simulink model "MPSKimparfait"  (Simulink 10.1)
settings: Solver=VariableStepAuto  StartTime=0.0  StopTime=inf  RelTol=1e-3
undefined symbols (not defined in the file or in its folder): M
libraries: commdigbbndpm3 x2, commfilt2 x2, commchan3 x1, commsync2 x1, commsink2 x1, commutil2 x1, commrflib2 x1, commrandsrc3 x1, dspsigops x1
settings Model: Creator=iba  LastModifiedBy=iba
settings DataIOCC: SaveFormat=Dataset  ReturnWorkspaceOutputs=on
settings OptimizationCC: LifeSpan=auto
settings DebuggingCC: UnderspecifiedInitializationDetection=Simplified  MergeDetectMultiDrivingBlocksExec=error  SFUnexpectedBacktrackingDiag=error  SFNoUnconditionalDefaultTransitionDiag=error  SFExecutionAtInitializationDiag=warning  ArithmeticOperatorsInVariantConditions=error
settings HardwareCC: ProdBitPerPointer=64  ProdBitPerSizeT=64  ProdBitPerPtrDiffT=64  ProdLargestAtomicFloat=Float  ProdIntDivRoundTo=Zero  ProdEndianess=LittleEndian  ProdWordSize=64  ProdHWDeviceType=Intel->x86-64 (Windows64)
settings ModelReferenceCC: PropagateSignalLabelsOutOfModel=on
settings SFSimCC: SimUseLocalCustomCode=on  CustomCodeUndefinedFunction=FilterOut
settings RTWCC: RTWUseLocalCustomCode=on
settings CodeAppCC: StateflowObjectComments=off
settings GRTTargetCC: TargetLangStandard=C99 (ISO)  CombineOutputUpdateFcns=on  GRTInterface=off
settings ConfigComp: CovMetricSettings=dwe  CovHtmlReporting=off  CovSaveCumulativeToWorkspaceVar=off  CovSaveSingleToWorkspaceVar=off  CovExternalEMLEnable=on

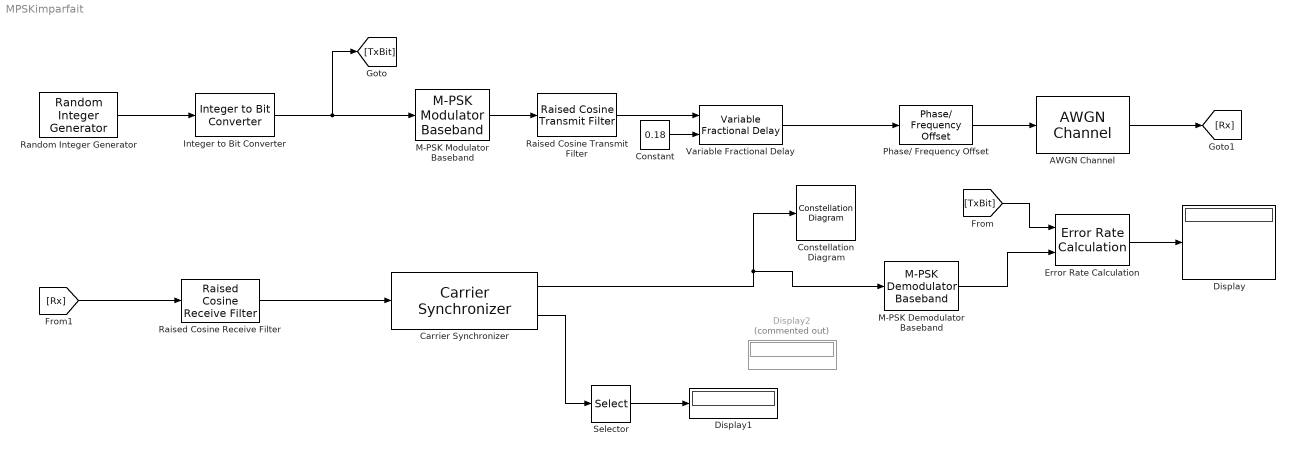
== system MPSKimparfait ==
  AWGN Channel : commchan3/AWGN Channel  InputProcessing=Columns as channels (frame based)  seed=67  noiseMode="Signal to noise ratio  (Eb/No)"  EbNodB=20  EsNodB=10  SNRdB=10  bitsPerSym=log2(M)  Ps=0.1  Tsym=1e-6  variance=1
  Carrier Synchronizer : commsync2/Carrier Synchronizer  Modulation=8PSK  ModulationPhaseOffset=Custom  CustomPhaseOffset=0  SamplesPerSymbol=1000  DampingFactor=0.701  NormalizedLoopBandwidth=0.0001  EstimatedPhaseErrorOutputPort=on  SimulateUsing=Code generation
  Constant : Constant  Value=0.18
  Constellation Diagram : ConstellationDiagram
  Display : Display
  Display1 : Display
  Display2 : Display  Commented=on
  Error Rate Calculation : commsink2/Error Rate Calculation  N=10*log2(M)  st_delay=0  cp_mode=Entire frame  subframe=[]  PMode=Port  WsName=MonTEB  RsMode2=off  stop=on  numErr=100  maxBits=1e6
  Integer to Bit Converter : commutil2/Integer to Bit Converter  nbits=log2(M)  signedInputValues=Unsigned  bitOrder=MSB first  outDtype=Inherit via internal rule
  M-PSK Demodulator Baseband : commdigbbndpm3/M-PSK Demodulator Baseband  M=M  OutType=Bit  DecType=Hard decision  VarSource=Dialog  Variance=1  Dec=Gray  Mapping=[0:7]  Ph=0  outDtype1=Inherit via internal rule  outDtype2=Inherit via internal rule  derotateFactorWordLen=16  derotateFactorDataTypeStr=Inherit: Same word length as input  derotateFactorLastDataTypeStr=Inherit: Same word length as input
  M-PSK Modulator Baseband : commdigbbndpm3/M-PSK Modulator Baseband  M=M  InType=Bit  Enc=Gray  Mapping=[0:7]  Ph=0  outDtype=double  outWordLen=16  outUDDataType=sfix(16)  outFracLenMode=Best precision  outFracLen=15  outDataTypeStr=double  outLastDataTypeStr=double
  Phase/ Frequency Offset : commrflib2/Phase// Frequency Offset  phaseOffset=18  freqPort=off  freqOffset=0
  Raised Cosine Receive Filter : commfilt2/Raised Cosine Receive Filter  filtType=Square root  R=0.7  filtSpan=10  N=10  downFactor=10  downOffset=0  filterGain=1  InputProcessing=Columns as channels (frame based)  RateOptions=Enforce single-rate processing  framing=Mute  checkCoeff=off  variableName=rcRxFilt  currentFiltSpan=10  D=(10)/2  inputOffset=0  sampMode=Mute  saveAsFlag=0  rateMode=Downsampling  checkGain=Normalized  launchFVT=on  roundingMode=Floor  overflowMode=off  coeffDataTypeStr=Inherit: Same word length as input  coeffMin=[]  coeffMax=[]  coeffLastDataTypeStr=Inherit: Same word length as input  accumDataTypeStr=Inherit: Same as product output  accumLastDataTypeStr=Inherit: Same as product output  outputDataTypeStr=Inherit: Same as accumulator  outputMin=[]  outputMax=[]  outputLastDataTypeStr=Inherit: Same as accumulator
  Raised Cosine Transmit Filter : commfilt2/Raised Cosine Transmit Filter  filtType=Square root  R=0.7  filtSpan=10  N=10  filterGain=1  InputProcessing=Columns as channels (frame based)  RateOptions=Enforce single-rate processing  framing=Mute  checkCoeff=off  variableName=rcTxFilt  checkGain=Normalized  sampMode=Mute  saveAsFlag=0  currentFiltSpan=10  D=5  launchFVT=on  roundingMode=Floor  overflowMode=off  coeffDataTypeStr=Inherit: Same word length as input  coeffMin=[]  coeffMax=[]  coeffLastDataTypeStr=Inherit: Same word length as input  outputDataTypeStr=Inherit: Same as accumulator  outputMin=[]  outputMax=[]  outputLastDataTypeStr=Inherit: Same as accumulator
  Random Integer Generator : commrandsrc3/Random Integer Generator  SetSize=M  SeedSource=Parameter  Seed=37  SampleTime=1e-6  SamplesPerFrame=1000  OutputDataType=double  SimulateUsing=Interpreted execution
  Selector : Selector  IndexOptions=Index vector (dialog)  Indices=1  OutputSizes=1
  Variable Fractional Delay : dspsigops/Variable Fractional Delay  mode=OBSOLETE  modeActive=Linear  L=4  FarrowL=4  R=10  alpha=1  dmax=10  InputProcessing=Columns as channels (frame based)  ic=0  noDFT=off  fallbackFIR=Clip to the minimum value necessary for centered kernel  fallbackFarrow=Clip to the minimum value necessary for centered kernel  roundingMode=Zero  overflowMode=off
      settings: SourceProductBaseCode=DS
  wires:
  Random Integer Generator/1 -> Integer to Bit Converter/1
  M-PSK Demodulator Baseband/1 -> Error Rate Calculation/2
  Raised Cosine Receive Filter/1 -> Carrier Synchronizer/1
  M-PSK Modulator Baseband/1 -> Raised Cosine Transmit Filter/1
  Integer to Bit Converter/1 -> [TxBit], M-PSK Modulator Baseband/1
  AWGN Channel/1 -> [Rx]
  [TxBit] -> Error Rate Calculation/1
  [Rx] -> Raised Cosine Receive Filter/1
  Error Rate Calculation/1 -> Display/1
  Raised Cosine Transmit Filter/1 -> Variable Fractional Delay/1
  Variable Fractional Delay/1 -> Phase/ Frequency Offset/1
  Constant/1 -> Variable Fractional Delay/2
  Carrier Synchronizer/2 -> Selector/1
  Selector/1 -> Display1/1
  Phase/ Frequency Offset/1 -> AWGN Channel/1
  Carrier Synchronizer/1 -> Constellation Diagram/1, M-PSK Demodulator Baseband/1
  ? -> Display2/1
